simulink model "ComplementaryFilterThetaEstimation"  (R2022b)
settings: Solver=VariableStepAuto  StartTime=0.0  StopTime=END  RelTol=1e-3
values from neighbouring files (symbols this model uses):
  biais_gyr = 1    [Set_Context_CFTE.m]
  freq = 0.25    [Set_Context_CFTE.m]
  g = 9.81    [Set_Context_CFTE.m]
  Ki = Kteta^2/4 - 1    (= 99)    [Set_Context_CFTE.m]
  Kteta = 20    [Set_Context_CFTE.m]
  sigma_acc = 0.022    [Set_Context_CFTE.m]
  sigma_gyr = 0.017    [Set_Context_CFTE.m]
  theta_max = 0.785398    [Set_Context_CFTE.m]
  Ts = 0.08    [Set_Context_CFTE.m]
undefined symbols (not defined in the file or in its folder): DiscIntNeverNeededParam
libraries: simulink x2, dspsrcs4 x1
settings Model: Creator=Hugo  LastModifiedBy=Hugo

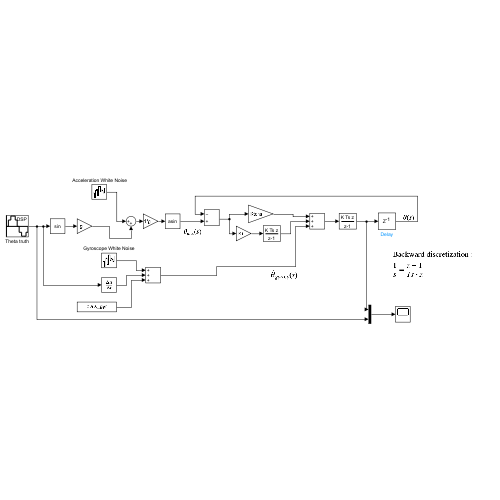
[thumbnail: Simulink's stored preview of the top-level diagram]
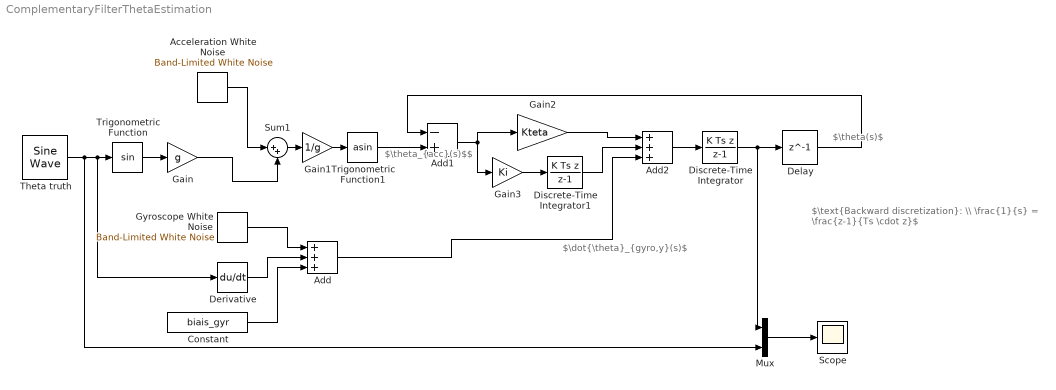
== system ComplementaryFilterThetaEstimation ==
  note: $\text{Backward discretization}: \\ \frac{1}{s} = \frac{z-1}{Ts \cdot z}$
  note: $\dot{\theta}_{gyro,y}(s)$
  note: $\theta_{acc}(s)$$
  note: $\theta(s)$
  " Acceleration White Noise" : simulink/Sources/Band-Limited White Noise  Cov=[sigma_acc]  Ts=Ts  seed=[23341]
  Add : Sum  Inputs=+++
  Add1 : Sum  Inputs=-+
  Add2 : Sum  Inputs=+++
  Constant : Constant  Value=biais_gyr
  Delay : Delay  DelayLength=1  InitialCondition=0
  Derivative : Derivative
  Discrete-Time Integrator : DiscreteIntegrator  IntegratorMethod=Integration: Backward Euler  SampleTime=-1  ICPrevOutput=DiscIntNeverNeededParam  ICPrevScaledInput=DiscIntNeverNeededParam
  Discrete-Time Integrator1 : DiscreteIntegrator  IntegratorMethod=Integration: Backward Euler  SampleTime=-1  ICPrevOutput=DiscIntNeverNeededParam  ICPrevScaledInput=DiscIntNeverNeededParam
  Gain : Gain  Gain=g
  Gain1 : Gain  Gain=1/g
  Gain2 : Gain  Gain=Kteta
  Gain3 : Gain  Gain=Ki
  Gyroscope White Noise : simulink/Sources/Band-Limited White Noise  Cov=[sigma_gyr]  Ts=Ts  seed=[23341]
  Mux : Mux  Inputs=2
  Scope : Scope
  Sum1 : Sum  Inputs=|++
  Theta truth : dspsrcs4/Sine Wave  Amplitude=theta_max  Frequency=freq  Phase=0  SampleMode=Discrete  OutComplex=Real  CompMethod=Trigonometric fcn  TableSize=Speed  SampleTime=1/1000  SamplesPerFrame=1  ResetState=Restart at time zero  OutputFrames=off  dataType=double  wordLen=16  udDataType=sfix(16)  fracBitsMode=Best precision  numFracBits=15  OutDataTypeStr=double  LastOutDataTypeStr=double
  Trigonometric Function : Trigonometry
  Trigonometric Function1 : Trigonometry  Operator=asin
  wires:
  Add2/1 -> Discrete-Time Integrator/1
  Discrete-Time Integrator/1 -> Mux/1, Delay/1
  Gain2/1 -> Add2/1
  Mux/1 -> Scope/1
  Theta truth/1 -> Mux/2, Derivative/1, Trigonometric Function/1
  Trigonometric Function/1 -> Gain/1
  " Acceleration White Noise"/1 -> Sum1/1
  Gain/1 -> Sum1/2
  Sum1/1 -> Gain1/1
  Gain1/1 -> Trigonometric Function1/1
  Add1/1 -> Gain2/1, Gain3/1
  Gain3/1 -> Discrete-Time Integrator1/1
  Discrete-Time Integrator1/1 -> Add2/2
  Gyroscope White Noise/1 -> Add/1
  Derivative/1 -> Add/2
  Constant/1 -> Add/3
  Delay/1 -> Add1/1
  Trigonometric Function1/1 -> Add1/2
  Add/1 -> Add2/3
